simulink model "mpcNoconstraint"  (R2020b)
settings: Solver=VariableStepAuto  StartTime=0.0  StopTime=20  FixedStep=0.01  RelTol=1e-3
values from neighbouring files (symbols this model uses):
  mpcSetting =     [mpcNoConstraint.mat]
  plantModel =     [mpcNoConstraint.mat]
undefined symbols (not defined in the file or in its folder): penaltyMatrix, sampletimeS
libraries: simulink x1
settings Model: Creator=yuto  LastModifiedBy=yuto

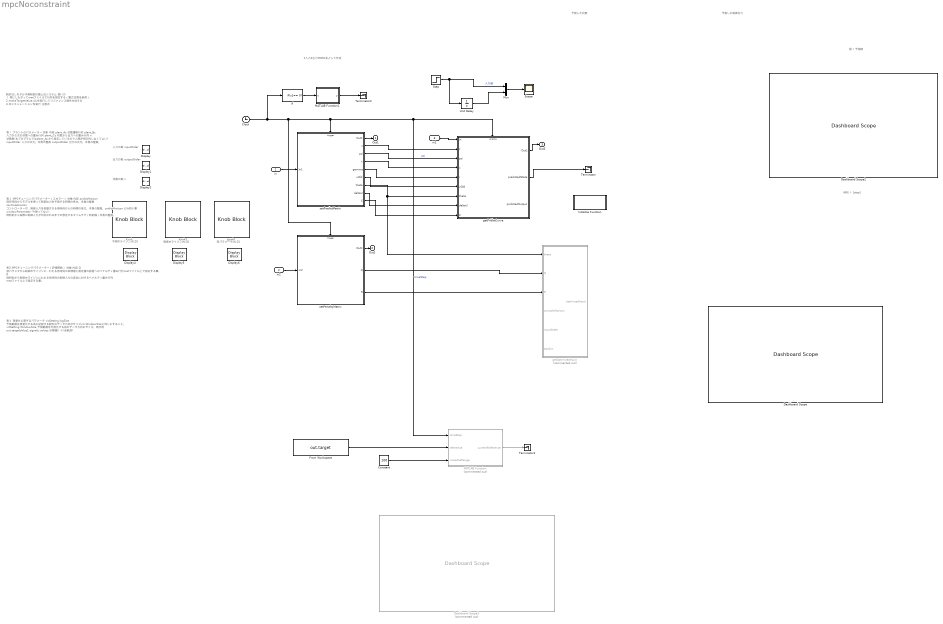
== system mpcNoconstraint ==
  note: 時刻 ｔ [step]
  note: 表４ 視覚化に関するパラメータ
      |
      | vizSetting.logSize
      | 予測範囲を視覚化する為に記録する配列のデータ方向のサイズviz.WindowSizeと同じにすること。
      |
      | vizSetting.WindowSize
      | 予測範囲を可視化する為のデータ方向のサイズ。表示用
      |
      | out.targetValue1.signals.values
      | 目標値ﾃﾞｰﾀ(全軌道)
  note: 予測した状態
  note: 予測ホライゾン[N,D]
  note: 入力の数
      | inputOrder
  note: 制約なしモデル予測制御の最上位システム
      | 使い方
      | １.表にしたがってmatファイルで行列を指定する（書式は表を参照）
      | 2.makeTargetValue.slxを実行してリファレンス値を生成する
      | 3.本シミュレーションを実行
      | 注意点
  note: 2入力2出力MIMO系として作成
  note: 表１ プラントのパラメーター
      | 対象
      | 内容
      |
      | plant_Ac
      | 状態遷移行列
      |
      | plant_Bc
      | 入力から次の状態への重み行列
      |
      | plant_Cy
      | 状態から出力への重み行列
      |
      | n
      | 状態数(本プログラムではplant_Acから指定しているので人間が明示的しなくてよい)
      |
      | inputOrder
      | 入力の次元。非負の整数
      |
      | outputOrder
      | 出力の次元。非負の整数。
  note: 表２ MPCチューニングパラメーター（スカラー）
      | 対象
      | 内容
      |
      | pridictHroizon
      | 現在時刻からモデルを使って制御出力を予測する時間の長さ。非負の整数
      |
      | controleHroizon
      | コントローラーが制御入力を変動させる現時刻からの時間の長さ。非負の整数。pridictHroizonよみ短い事
      |
      | windowParameter
      | (今使ってない)
      | 現時刻から実際に制御入力が印加されるまでの想定するタイムラグ（時刻幅）非負の整数。
  note: 表3 MPCチューニングパラメーター（評価関数）
      | 対象
      | 内容
      |
      | Q
      | 窓パラメタから制御ホライゾンにわたる各時刻の目標値と測定値の誤差へのペナルティ重み行列matファイル上で指定する事。
      |
      | R
      | 現時刻から制御ホライゾンにわたる各時刻の制御入力の変位に対するペナルティ重み行列
      | matファイル上で指定する事。
  note: 出力の数
      | outputOrder
  note: 状態の数
      | n
  note: 制御ホライゾン[N,D]
  note: 窓パラメータ[N,D]
  note: 予測した制御出力
  note: 図１ 予測線
  in : Inport
  in2 : Inport  Port=2
  in1 : Inport  Port=3
  Clock : Clock
  Constant : Constant  Value=100
  Dashboard Scope : DashboardScope  TimeSpan=20  Ymin=-2  LegendPosition=Hide  ScaleAtStop=off
  Dashboard Scope2 : DashboardScope  TimeSpan=20  Ymin=-2  LegendPosition=Hide
  Dashboard Scope3 : DashboardScope  Commented=on  TimeSpan=20  Ymin=-2  LegendPosition=Hide
  Display{,1..2,4..6} (6 alike) : DisplayBlock  LabelPosition=Hide  Format=short  Transparency=1
  From Workspace : FromWorkspace  VariableName=out.target
  If : If  IfExpression=u1== 0  ShowElse=off
  Initialize Function : Subsystem  TreatAsAtomicUnit=on
  Knob : KnobBlock  LabelPosition=Hide  ScaleMax=25  TickInterval=5
  Knob1 : KnobBlock  LabelPosition=Hide  ScaleMax=50  TickInterval=10
  Knob2 : KnobBlock  LabelPosition=Hide  ScaleMax=50  TickInterval=10
  MATLAB Function : MATLAB Function  Commented=on  TreatAsAtomicUnit=on
  MATLAB Function1 : MATLAB Function  TreatAsAtomicUnit=on
  Mux : Mux  Inputs=2
  Scope : Scope
  Step : Step  SampleTime=0
  Terminator : Terminator
  Terminator1 : Terminator
  Terminator2 : Terminator
  Unit Delay : UnitDelay  SampleTime=-1  HasFrameUpgradeWarning=on
  getOptimizedInput : MATLAB Function  Commented=on  TreatAsAtomicUnit=on
  getPridictCurve : Subsystem  TreatAsAtomicUnit=on
      mask Display: image('C:\Users\yuto\Documents\matlab\mpcNoConstraint\03_icons\predictCurveIcon.png'); % 変更するには、ツールストリップの [イメージの編集] を使用してください。
  setPenaltyMatrix : Subsystem  TreatAsAtomicUnit=on
      mask Display: image('C:\Users\yuto\Documents\matlab\mpcNoConstraint\03_icons\penaltyMatrixSettingicon.png'); % 変更するには、ツールストリップの [イメージの編集] を使用してください。
  setPredictMatrix : Subsystem  TreatAsAtomicUnit=on
      mask Display: image('C:\Users\yuto\Documents\matlab\mpcNoConstraint\03_icons\predectMatrixSettingicon.png'); % 変更するには、ツールストリップの [イメージの編集] を使用してください。
  Out1 : Outport
  Out2 : Outport  Port=2
  Out3 : Outport  Port=3
  wires:
  in/1 -> setPredictMatrix/1(In1)
  getPridictCurve/2(predictedState) -> Terminator/1
  in2/1 -> setPenaltyMatrix/1(in2)
  setPredictMatrix/8(deltaU) -> getPridictCurve/8(deltaU)
  setPredictMatrix/7(theta) -> getOptimizedInput/1(theta), getPridictCurve/7(theta)
  setPredictMatrix/6(uOld) -> getPridictCurve/6(uOld)
  setPredictMatrix/5(gamma) -> getPridictCurve/5(r)
  setPredictMatrix/4(x) -> getPridictCurve/4(x)
  setPredictMatrix/3(psi) -> getPridictCurve/3(psi)  "psi"
  setPredictMatrix/2(z) -> getPridictCurve/2(z)
  setPenaltyMatrix/2(Q) -> getOptimizedInput/2(Q)
  setPenaltyMatrix/3(R) -> getOptimizedInput/3(R)
  setPredictMatrix/1(Out1) -> Out1/1
  setPenaltyMatrix/1(Out1) -> Out2/1
  setPredictMatrix/9(C) -> getPridictCurve/9(C)
  getPridictCurve/1(Out1) -> Out3/1
  in1/1 -> getPridictCurve/1(in)
  Clock/1 -> If/1, MATLAB Function/1(timeStep), getPridictCurve/Enable, setPredictMatrix/Trigger, setPenaltyMatrix/Trigger  "timeStep"
  From Workspace/1 -> MATLAB Function/2(reference)
  MATLAB Function/1(currentReference) -> Terminator1/1
  Constant/1 -> MATLAB Function/3(visualizeRange)
  Step/1 -> Unit Delay/1, Mux/1  "入力値"
  Unit Delay/1 -> Mux/2
  Mux/1 -> Scope/1
  If/1 -> MATLAB Function1/1(u)
  MATLAB Function1/1(y) -> Terminator2/1

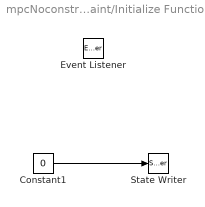
== system mpcNoconstraint/Initialize Function ==
  Constant1 : Constant  Value=0
  Event Listener : EventListener  DisableCoverage=on  EventName=reset
  State Writer : StateWriter
  wires:
  Constant1/1 -> State Writer/1

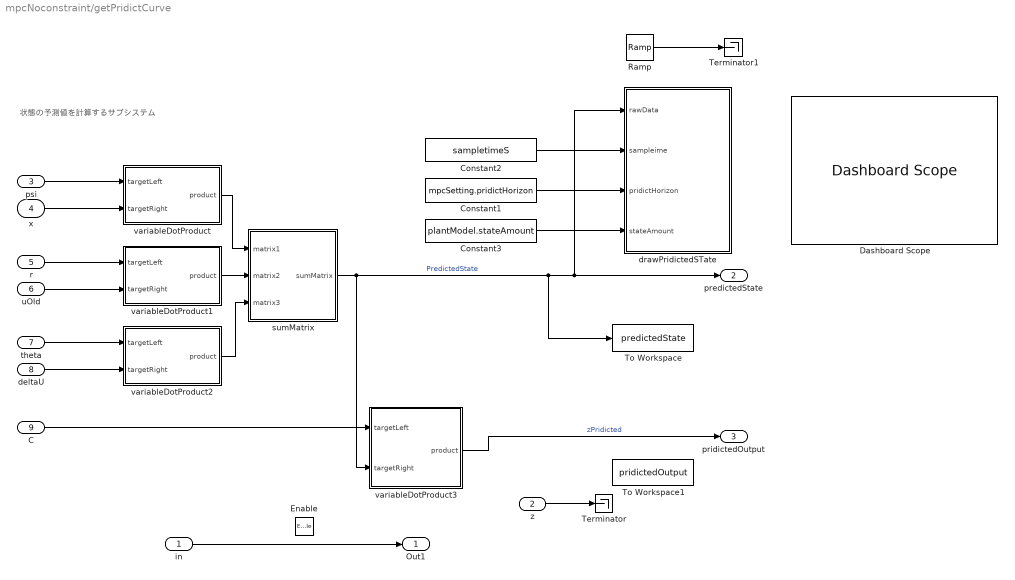
== system mpcNoconstraint/getPridictCurve ==
  note: 状態の予測値を計算するサブシステム
  in : Inport
  z : Inport  Port=2
  psi : Inport  Port=3
  x : Inport  Port=4
  r : Inport  Port=5
  uOld : Inport  Port=6
  theta : Inport  Port=7  SampleTime=[sampletimeS 0]
  deltaU : Inport  Port=8
  C : Inport  Port=9
  Enable : EnablePort  PropagateVarSize=During execution
  Constant1 : Constant  Value=mpcSetting.pridictHorizon
  Constant2 : Constant  Value=sampletimeS
  Constant3 : Constant  Value=plantModel.stateAmount
  Dashboard Scope : DashboardScope
  Ramp : simulink/Sources/Ramp  slope=1  start=0  InitialOutput=0
  Terminator : Terminator
  Terminator1 : Terminator
  To Workspace : ToWorkspace  VariableName=predictedState  SaveFormat=Structure With Time  SampleTime=-1
  To Workspace1 : ToWorkspace  VariableName=pridictedOutput  SaveFormat=Structure With Time  SampleTime=-1
  drawPridictedSTate : MATLAB Function  TreatAsAtomicUnit=on
  sumMatrix : MATLAB Function  TreatAsAtomicUnit=on
  variableDotProduct : MATLAB Function  TreatAsAtomicUnit=on  SystemSampleTime=sampletimeS
  variableDotProduct1 : MATLAB Function  TreatAsAtomicUnit=on  SystemSampleTime=sampletimeS
  variableDotProduct2 : MATLAB Function  TreatAsAtomicUnit=on  SystemSampleTime=sampletimeS
  variableDotProduct3 : MATLAB Function  TreatAsAtomicUnit=on  SystemSampleTime=0.1
  Out1 : Outport
  predictedState : Outport  Port=2
  pridictedOutput : Outport  Port=3
  wires:
  in/1 -> Out1/1
  uOld/1 -> variableDotProduct1/2(targetRight)
  psi/1 -> variableDotProduct/1(targetLeft)
  sumMatrix/1(sumMatrix) -> variableDotProduct3/2(targetRight), To Workspace/1, drawPridictedSTate/1(rawData), predictedState/1  "PredictedState"
  variableDotProduct/1(product) -> sumMatrix/1(matrix1)
  x/1 -> variableDotProduct/2(targetRight)
  deltaU/1 -> variableDotProduct2/2(targetRight)
  r/1 -> variableDotProduct1/1(targetLeft)
  z/1 -> Terminator/1
  variableDotProduct1/1(product) -> sumMatrix/2(matrix2)
  variableDotProduct2/1(product) -> sumMatrix/3(matrix3)
  variableDotProduct3/1(product) -> pridictedOutput/1  "zPridicted"
  C/1 -> variableDotProduct3/1(targetLeft)
  theta/1 -> variableDotProduct2/1(targetLeft)
  Constant2/1 -> drawPridictedSTate/2(sampleime)
  Ramp/1 -> Terminator1/1
  Constant1/1 -> drawPridictedSTate/3(pridictHorizon)
  Constant3/1 -> drawPridictedSTate/4(stateAmount)

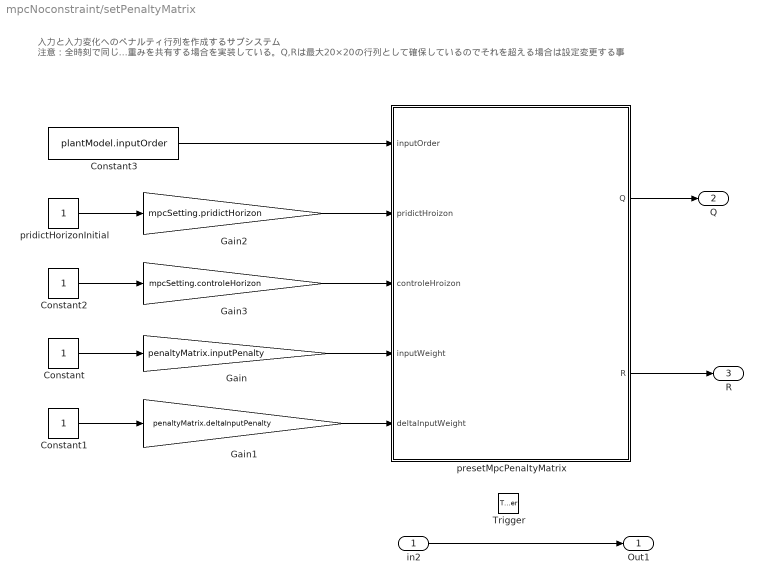
== system mpcNoconstraint/setPenaltyMatrix ==
  note: 入力と入力変化へのペナルティ行列を作成するサブシステム
      |
      | 注意：全時刻で同じ重みを共有する場合を実装している。Q,Rは最大20×20の行列として確保しているのでそれを超える場合は設定変更する事
  in2 : Inport
  Trigger : TriggerPort  VariantControl=Variant
  Constant : Constant
  Constant1 : Constant
  Constant2 : Constant
  Constant3 : Constant  Value=plantModel.inputOrder
  Gain : Gain  Gain=penaltyMatrix.inputPenalty
  Gain1 : Gain  Gain=penaltyMatrix.deltaInputPenalty
  Gain2 : Gain  Gain=mpcSetting.pridictHorizon
  Gain3 : Gain  Gain=mpcSetting.controleHorizon
  presetMpcPenaltyMatrix : MATLAB Function  TreatAsAtomicUnit=on
  pridictHorizonInitial : Constant
  Out1 : Outport
  Q : Outport  Port=2
  R : Outport  Port=3
  wires:
  in2/1 -> Out1/1
  Gain3/1 -> presetMpcPenaltyMatrix/3(controleHroizon)
  Gain2/1 -> presetMpcPenaltyMatrix/2(pridictHroizon)
  Constant3/1 -> presetMpcPenaltyMatrix/1(inputOrder)
  presetMpcPenaltyMatrix/2(R) -> R/1
  presetMpcPenaltyMatrix/1(Q) -> Q/1
  Gain/1 -> presetMpcPenaltyMatrix/4(inputWeight)
  Constant/1 -> Gain/1
  Constant1/1 -> Gain1/1
  Gain1/1 -> presetMpcPenaltyMatrix/5(deltaInputWeight)
  pridictHorizonInitial/1 -> Gain2/1
  Constant2/1 -> Gain3/1

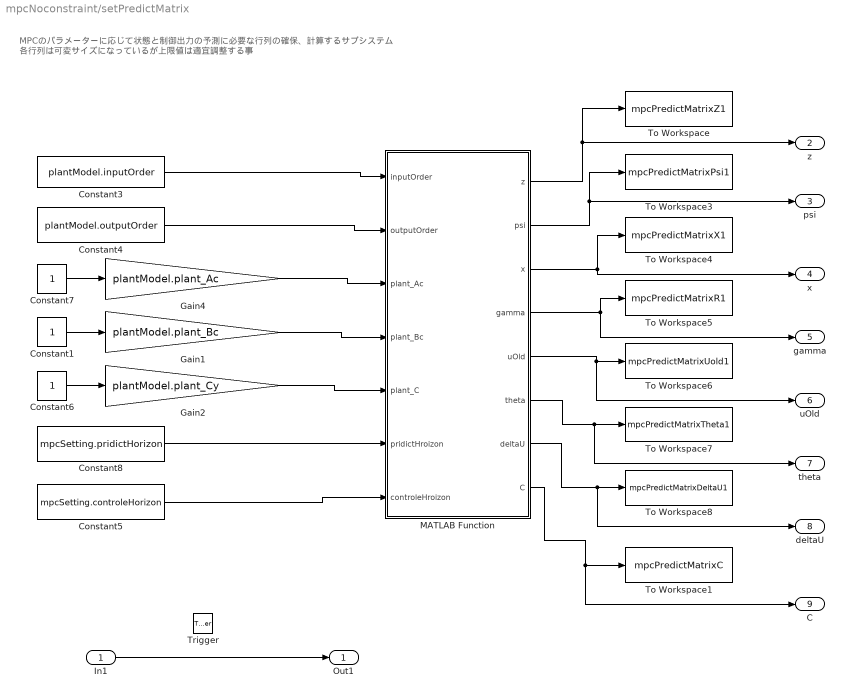
== system mpcNoconstraint/setPredictMatrix ==
  note: MPCのパラメーターに応じて状態と制御出力の予測に必要な行列の確保、計算するサブシステム
      | 各行列は可変サイズになっているが上限値は適宜調整する事
  In1 : Inport
  Trigger : TriggerPort  VariantControl=Variant
  Constant1 : Constant
  Constant3 : Constant  Value=plantModel.inputOrder
  Constant4 : Constant  Value=plantModel.outputOrder
  Constant5 : Constant  Value=mpcSetting.controleHorizon  SampleTime=-1
  Constant6 : Constant
  Constant7 : Constant
  Constant8 : Constant  Value=mpcSetting.pridictHorizon  SampleTime=-1
  Gain1 : Gain  Gain=plantModel.plant_Bc
  Gain2 : Gain  Gain=plantModel.plant_Cy
  Gain4 : Gain  Gain=plantModel.plant_Ac
  MATLAB Function : MATLAB Function  TreatAsAtomicUnit=on
  To Workspace : ToWorkspace  VariableName=mpcPredictMatrixZ1  SaveFormat=Structure  SampleTime=-1
  To Workspace1 : ToWorkspace  VariableName=mpcPredictMatrixC  SaveFormat=Structure With Time  SampleTime=-1
  To Workspace3 : ToWorkspace  VariableName=mpcPredictMatrixPsi1  SaveFormat=Structure  SampleTime=-1
  To Workspace4 : ToWorkspace  VariableName=mpcPredictMatrixX1  SaveFormat=Structure With Time  SampleTime=-1
  To Workspace5 : ToWorkspace  VariableName=mpcPredictMatrixR1  SaveFormat=Structure  SampleTime=-1
  To Workspace6 : ToWorkspace  VariableName=mpcPredictMatrixUold1  SaveFormat=Structure With Time  SampleTime=-1
  To Workspace7 : ToWorkspace  VariableName=mpcPredictMatrixTheta1  SaveFormat=Structure  SampleTime=-1
  To Workspace8 : ToWorkspace  VariableName=mpcPredictMatrixDeltaU1  SaveFormat=Structure With Time  SampleTime=-1
  Out1 : Outport
  z : Outport  Port=2
  psi : Outport  Port=3
  x : Outport  Port=4
  gamma : Outport  Port=5
  uOld : Outport  Port=6
  theta : Outport  Port=7
  deltaU : Outport  Port=8
  C : Outport  Port=9
  wires:
  In1/1 -> Out1/1
  Gain1/1 -> MATLAB Function/4(plant_Bc)
  Constant6/1 -> Gain2/1
  Gain2/1 -> MATLAB Function/5(plant_C)
  MATLAB Function/7(deltaU) -> deltaU/1, To Workspace8/1
  Gain4/1 -> MATLAB Function/3(plant_Ac)
  MATLAB Function/2(psi) -> To Workspace3/1, psi/1
  MATLAB Function/4(gamma) -> To Workspace5/1, gamma/1
  MATLAB Function/5(uOld) -> uOld/1, To Workspace6/1
  Constant4/1 -> MATLAB Function/2(outputOrder)
  MATLAB Function/3(x) -> To Workspace4/1, x/1
  Constant1/1 -> Gain1/1
  Constant3/1 -> MATLAB Function/1(inputOrder)
  MATLAB Function/6(theta) -> theta/1, To Workspace7/1
  MATLAB Function/1(z) -> To Workspace/1, z/1
  Constant5/1 -> MATLAB Function/7(controleHroizon)
  MATLAB Function/8(C) -> C/1, To Workspace1/1
  Constant7/1 -> Gain4/1
  Constant8/1 -> MATLAB Function/6(pridictHroizon)

== matlab function mpcNoconstraint/getPridictCurve/sumMatrix ==
  data: matrix1 input size=[mpcSetting.pridictHorizon*plantModel.stateAmount 1]; matrix2 input size=[mpcSetting.pridictHorizon*plantModel.stateAmount 1]; sumMatrix output size=[mpcSetting.pridictHorizon*plantModel.stateAmount 1]; matrix3 input size=[mpcSetting.pridictHorizon*plantModel.stateAmount 1]
function sumMatrix = fcn(matrix1,matrix2,matrix3)

    %% 可変行列の為に自前で行列和計算を計算
%全ての入力行列のサイズが揃っている事が前提条件
    % 和計算結果行列の定義
    sumMatrix = zeros(size(matrix1,1),size(matrix1,2));
    
    % 行についてのループ計算
    for i = 1:1:size(matrix1,1)
       
        % 列についての要素ループ
        for j = 1:1:size(matrix1,2)
            
            % 各要素の和を計算
            sumMatrix(i,j) = matrix1(i,j) + matrix2(i,j) + matrix3(i,j);
            
        end
        
    end

end

== matlab function mpcNoconstraint/getPridictCurve/drawPridictedSTate ==
  data: rawData input size=[plantModel.stateAmount*mpcSetting.pridictHorizon 1]; sampleime input; pridictHorizon input; stateAmount input
function drawPridictedAmount(rawData, sampleime, pridictHorizon,stateAmount)

    % このファイルを外部のものとして定義
    coder.extrinsic('drawPredictedAmounts.m');
    
    % figオブジェクトの永続変数として作成
    persistent call;
    
    % 初回の呼び出しかを判断
    if isempty(call)
        
        % 永続変数を０でリセット
        call = 0;
        
        % 時間軸(現在から未来への相対的な時間)のデータを作成  
        time = linspace(0,pridictHorizon*sampleime,pridictHorizon);
       
        % 値を生データから取り出すインデックスベクトルの作成
        valueIndex = linspace(1,size(rawData,1),pridictHorizon / stateAmount);
        
        % 確認表示
        disp('current call Index');
        disp(call);
        disp('time vector');
        disp();
        disp('value vector');
        disp(valueIndex);
        
        % 状態の数だけ別々にfigオブジェクトを作成
        for figIndex = 1:stateAmount
            figure(figIndex);
        end
        
        for stateIndex = 1:stateAmount

            % グリッドの表示
            grid on
            
            % 軸の設定
            axis([0 5 -5 5]);
            
            % ある１つの状態をプロットする処理
           plot(time,rawData(valueIndex));
            

        end
    else

    end
    
    % 永続変数をインクリメントする
    call = call + 1;

end

== matlab function mpcNoconstraint/MATLAB Function1 ==
  data: u input; y output
function y = reset(u)
sim('makeTargetValue.slx');
y = u;
end

== matlab function mpcNoconstraint/getPridictCurve/variableDotProduct3 ==
  data: targetLeft input size=[plantModel.outputOrder*mpcSetting.pridictHorizon mpcSetting.pridictHorizon*plantModel.stateAmount]; targetRight input size=[mpcSetting.pridictHorizon*plantModel.stateAmount 1]; product output size=[mpcSetting.pridictHorizon*plantModel.outputOrder 1]
function product = fcn(targetLeft,targetRight)

    %% 可変行列の為に自前で外積計算を書く関数

    % 外積計算結果行列の定義
    product = zeros(size(targetLeft,1),size(targetRight,2));
    for i = 1:1:size(targetLeft,1)
       
        for j = 1:1:size(targetRight,2)
        
            tmp = 0;
            for k = 1:1:size(targetRight,1)
                tmp = tmp + targetRight(k,j);
            end
            product(i,j) = tmp;
        end
        
    end


end

== matlab function mpcNoconstraint/MATLAB Function ==
  data: timeStep input; currentReference output size=[100 2]; reference input; visualizeRange input

function currentReference   = fcn(timeStep,reference,visualizeRange)

    % 参照値保存用配列の確保　一時的に０で埋める
    currentReference = zeros(visualizeRange,2);
    
    % 参照値（現在は目標値そのままとする）を表す行列を作成　1行目が下に向かって時刻ステップ　列方向が値 現在1変数のみ対応
    tmp = reference(timeStep:timeStep + visualizeRange);
    
    % 現在からの相対的な
    index = ones(visualizeRange,1);
   % 各時刻の参照値の行列を作成
   currentReference =[index tmp];
    
    
end

== matlab function mpcNoconstraint/setPredictMatrix/MATLAB Function ==
  data: inputOrder input; outputOrder input; plant_Ac input size=[size(plantModel.plant_Ac)]; plant_Bc input; plant_C input; pridictHroizon input; z output size=[mpcSetting.pridictHorizon*plantModel.stateAmount   plantModel.stateAmount]; psi output size=[mpcSetting.pridictHorizon*plantModel.stateAmount   plantModel.stateAmount]; controleHroizon input; x output size=[plantModel.stateAmount 1]; gamma output size=[mpcSetting.pridictHorizon*plantModel.stateAmount plantModel.inputOrder]; uOld output size=[plantModel.inputOrder 1]; theta output size=[mpcSetting.pridictHorizon*plantModel.stateAmount mpcSetting.controleHorizon*plantModel.inputOrder]; deltaU output size=[mpcSetting.controleHorizon*plantModel.inputOrder 1]; C output size=[mpcSetting.pridictHorizon*plantModel.outputOrder mpcSetting.pridictHorizon*plantModel.stateAmount]
function [z,psi,x,gamma,uOld,theta,deltaU,C] = presetPredictMatrix(inputOrder,outputOrder,plant_Ac,plant_Bc,plant_C,pridictHroizon ,controleHroizon)

   %% 各種行列を確保する
   
   %状態の予測値行列zの作成　各要素は仮　注意！予測器が動的に変化する場合ここでの初期化処理を削除する必要がある
   z = zeros((size(plant_Ac,1) * pridictHroizon),1,'double');

   % 現在の状態から予測ホライゾンまでの先の状態への重み行列プサイのメモリを確保要素は仮
   psi = zeros(size(plant_Ac,1) * pridictHroizon,size(plant_Ac,2),'double');

   % 現在の状態を表す行列x(k)のメモリを確保要素は仮　注意！予測器が動的に変化する場合ここでの初期化処理を削除する必要がある
   x = zeros(size(plant_Ac,1),1,'double');
  
   % 1ステップ前の入力から予測ホライゾンまでの先の状態への重み行列ｒのメモリを確保要素は仮
   gamma = zeros((size(plant_Ac,1) * pridictHroizon),inputOrder,'double');
  
   % 1ステップ前の入力かu(k-1)のメモリを確保要素は仮
   uOld = zeros(inputOrder,1,'double');
  
   % 未来の入力変化から予測ホライゾンまでの先の状態への重み行列Θのメモリを確保要素は仮
   theta= zeros((size(plant_Ac,1) * pridictHroizon),(controleHroizon * inputOrder),'double');
  
   % 未来の入力変化行列deltaUのメモリを確保要素は仮
   deltaU= zeros((controleHroizon * inputOrder),1,'double');
  
   % 状態から出力へのぎょるえつのメモリを確保要素は仮
   C = zeros((pridictHroizon * outputOrder),(pridictHroizon * size(plant_Ac,1)),'double');
  
  %作成された行列のサイズを確認表示
  disp('gamma size');
  disp(size(gamma,1));
  disp(size(gamma,2));
  
  disp(size(theta,1));
  disp(size(theta,2));
  
  disp(size(C,1));
  disp(size(C,2));
  
  %% 行列プサイの内容を求める
  
   % 行方向へのＡの行数ごとのループ
   for i = 1: pridictHroizon
       
       % 行列Aの累乗を計算
        tmp = power(plant_Ac,i);
        
        % 計算結果を行列プサイの適切な箇所に格納
        psi((i - 1) * size(plant_Ac,1) + 1 :i * size(plant_Ac,1),1: size(plant_Ac,2)) = tmp;
      
   end
   
   %% 入力から予測状態への重み行列γの作成
    
   % 行方向へのＡの行数ごとのループ
   for i = 1:pridictHroizon
       
       if i == 1
      
            %B行列を結果として行列ｒの適切な部分へ格納 size(plant_Bc,2)
            gamma(1:size(plant_Bc,1),1:inputOrder) = plant_Bc(1:size(plant_Bc,1),1:size(plant_Bc,2));
            
            % 確認表示
            %disp(gamma(1:size(plant_Bc,1),1:size(plant_Bc,2)));
           
       else
            powerdA =  power(plant_Ac,(i-1));
             
            % A累乗行列とBの外積行列を結果として行列ｒの適切な部分へ格納
            gamma((i - 1) * size(plant_Ac,1) + 1 :i * size(plant_Ac,1),1: size(plant_Bc,2)) =  powerdA * plant_Bc;
            
            % 確認表示
            %disp(gamma((i - 1) * size(plant_Ac,1) + 1 :i * size(plant_Ac,1),1: size(plant_Bc,2)));
       end
   end
   
   %% 未来の入力変化から予測した状態への重み行列Θを求める
   
   % 行についての状態数ごとのループ
    for i = 1:pridictHroizon
   
        % 列についての入力数ごとのループ
        for j = 1:controleHroizon

            if j < i
        
                %　生成行列一時保存用行列の確保
                tmp = zeros(size(plant_Ac,1),size(plant_Bc,2));
            
                % Θ行列対角要素より下の要素の計算に必要なΣ計算用forループ
                for k = 1:(i - j)
                    tmp = power(plant_Ac,k) * plant_Bc;
                end
                element = tmp + plant_Bc;
                
                % 対角成分より下の要素の計算結果を代入
                theta((i - 1) * size(plant_Ac,1) + 1 :i * size(plant_Ac,1),((j - 1) * size(plant_Bc,2) + 1 ): j * size(plant_Bc,2))  = element;
           
            elseif i == j
                
                % 対角成分はB（A^0＝Bとならないのでこのように表記）（０乗が単位行列じゃないので）
                theta((i - 1) * size(plant_Ac,1) + 1 :i * size(plant_Ac,1),((j - 1) * size(plant_Bc,2) + 1 ): j * size(plant_Bc,2)) =plant_Bc;
            end
       end
    end
    
    %% 状態から出力への係数行列Cの内容を作成する
    
    for i= 1:pridictHroizon
        
       % 計算結果を行列Cの適切な箇所に格納 todo
       %C((i - 1) * size(plant_C,1) + 1 :i * size(plant_C,1),((i - 1) * size(plant_C,2) + 1 ): (i - 1) * size(plant_C,2)) = plant_C;
    end
       
    disp(C)
end

== matlab function mpcNoconstraint/setPenaltyMatrix/presetMpcPenaltyMatrix ==
  data: inputOrder input; Q output size=[20 20]; pridictHroizon input; controleHroizon input; R output size=[20 20]; inputWeight input; deltaInputWeight input
function [Q,R] = presetMpcPenaltyMatrix(inputOrder,pridictHroizon ,controleHroizon,inputWeight,deltaInputWeight)

    % 重み行列Qを確保
    Q = zeros(size(inputWeight,1) * (pridictHroizon - controleHroizon + 1),size(inputWeight,2) * (pridictHroizon - controleHroizon + 1));
    
    % 重み行列Rを確保
    R = zeros(inputOrder * controleHroizon,inputOrder * controleHroizon);
    
    % 行列Qの内容を作る
    for i = 1: 1:(pridictHroizon - controleHroizon + 1)
        
        Q( ( i - 1 ) * size(inputWeight,1) + 1: i * size(inputWeight,1),(i - 1) * size(inputWeight,2) + 1: i * size(inputWeight,2)) = inputWeight;
    end
    
    % 行列Rの内容を作る
    for i = 1: 1:controleHroizon
        
      %R( ( i - 1 ) * size(deltaInputWeight,1) + 1: i * size(deltaInputWeight,1),(i - 1) * size(deltaInputWeight,2) + 1: i * size(deltaInputWeight,2)) = deltaInputWeight;
        
    end
end

== matlab function mpcNoconstraint/getPridictCurve/variableDotProduct ==
  data targetLeft settings: description=プラントのシステム行列の累乗が格納された行列
  data targetRight settings: description=状態を示すベクトル
  data product settings: description=プラントのシステム行列の累乗の行列とプラントの状態ベクトルの外積結果を示す行列
  data: targetLeft input size=[mpcSetting.pridictHorizon*plantModel.stateAmount   plantModel.stateAmount]; targetRight input size=[plantModel.stateAmount 1]; product output size=[mpcSetting.pridictHorizon*plantModel.stateAmount 1]
function product = fcn(targetLeft,targetRight)

    %% 可変行列の為に自前で外積計算を書く関数

    % 外積計算結果行列の定義
    product = zeros(size(targetLeft,1),size(targetRight,2));
    for i = 1:1:size(targetLeft,1)
       
        for j = 1:1:size(targetRight,2)
        
            tmp = 0;
            for k = 1:1:size(targetRight,1)
                tmp = tmp + targetRight(k,j);
            end
            product(i,j) = tmp;
        end
        
    end


end

== matlab function mpcNoconstraint/getPridictCurve/variableDotProduct1 ==
  data targetRight settings: description=1ステップ前の入力
  data: targetLeft input size=[mpcSetting.pridictHorizon*plantModel.stateAmount plantModel.inputOrder]; targetRight input size=[plantModel.inputOrder 1]; product output size=[mpcSetting.pridictHorizon*plantModel.stateAmount 1]
function product = fcn(targetLeft,targetRight)

    %% 可変行列の為に自前で外積計算を書く関数

    % 外積計算結果行列の定義
    product = zeros(size(targetLeft,1),size(targetRight,2));
    for i = 1:1:size(targetLeft,1)
       
        for j = 1:1:size(targetRight,2)
        
            tmp = 0;
            for k = 1:1:size(targetRight,1)
                tmp = tmp + targetRight(k,j);
            end
            product(i,j) = tmp;
        end
        
    end


end

== matlab function mpcNoconstraint/getPridictCurve/variableDotProduct2 ==
  data: targetLeft input size=[mpcSetting.pridictHorizon*plantModel.stateAmount mpcSetting.controleHorizon*plantModel.inputOrder]; targetRight input size=[mpcSetting.controleHorizon*plantModel.inputOrder 1]; product output size=[mpcSetting.pridictHorizon*plantModel.stateAmount 1]
function product = fcn(targetLeft,targetRight)

    %% 可変行列の為に自前で外積計算を書く関数

    % 外積計算結果行列の定義
    product = zeros(size(targetLeft,1),size(targetRight,2));
    for i = 1:1:size(targetLeft,1)
       
        for j = 1:1:size(targetRight,2)
        
            tmp = 0;
            for k = 1:1:size(targetRight,1)
                tmp = tmp + targetRight(k,j);
            end
            product(i,j) = tmp;
        end
        
    end


end

== matlab function mpcNoconstraint/getOptimizedInput ==
  data: theta input; Q input; R input; optimizedInput output; controleHorizon input; inputOrder input; epsilon input
function optimizedInput = fcn(theta,Q,R,controleHorizon,inputOrder,epsilon)

    % 最適制御入力ベクトルを作成する関数
    % 逆行列から求める最もシンプルな方法だが行列が悪条件になるのでこの処理は仮　将来的に置き換え予定
    
    % 行列ｇを作成
    g = zeros( inputOrder * controleHorizon,1,'double');
    
    % 行列Ｈを作成
    H = zeros( inputOrder * controleHorizon ,inputOrder * controleHorizon,'double');
    
    % 行列gを計算
    g = 2 * transepose(theta) * Q * epsilon;
    
    % 行列Hを計算
    H = transepose(theta) * Q * theta + R;
    
    % delta
end
